simulink model "SvSDP_SimModel_FINAL_REV0"  (R2016b)
settings: Solver=ode3  StartTime=0  StopTime=15  FixedStep=T_sim  MaxStep=0.001  RelTol=1e-3  EnableMultiTasking=on
values from neighbouring files (symbols this model uses):
  A_A = pi/4*Dp^2    (= 0.00311724531052)    [par_SvSDP_SimModel_FINAL_REV0.m]
  A_B = pi/4*(Dp^2-Dr^2)    (= 0.00215513256036)    [par_SvSDP_SimModel_FINAL_REV0.m]
  beta_F = 7500e5    (= 750000000)    [par_SvSDP_SimModel_FINAL_REV0.m]
  Bs = 6480    [par_SvSDP_SimModel_FINAL_REV0.m]
  Drive_lim_max = 3000*pi/30    (= 314.159265359)    [par_SvSDP_SimModel_FINAL_REV0.m]
  Drive_lim_min = -3000*pi/30    (= -314.159265359)    [par_SvSDP_SimModel_FINAL_REV0.m]
  Drive_v_lim = 95e3*pi/30    (= 9948.37673637)    [par_SvSDP_SimModel_FINAL_REV0.m]
  dx_stribeck = 7e-3    (= 0.007)    [par_SvSDP_SimModel_FINAL_REV0.m]
  eta_air = 0.7e-2    (= 0.007)    [par_SvSDP_SimModel_FINAL_REV0.m]
  Fcs = 1740.8    [par_SvSDP_SimModel_FINAL_REV0.m]
  Fext = 20e3    (= 20000)    [par_SvSDP_SimModel_FINAL_REV0.m]
  Fss = Fcs+50    (= 1790.8)    [par_SvSDP_SimModel_FINAL_REV0.m]
  gammas = 1700    [par_SvSDP_SimModel_FINAL_REV0.m]
  I_nomK100 = 15.8    [par_SvSDP_SimModel_FINAL_REV0.m]
  Kad = H/(H+alpha)^2*abs(K_LpL)*10000    [par_SvSDP_SimModel_FINAL_REV0.m]
  kappa_air = 1.4    [par_SvSDP_SimModel_FINAL_REV0.m]
  kn_ad = A_A*(H+alpha)^2/(A_A^2*(H+alpha)^2+Bs*H*(K_LpL+Kad))    [par_SvSDP_SimModel_FINAL_REV0.m]
  Ms = 658    [par_SvSDP_SimModel_FINAL_REV0.m]
  pA_ini = Fext/A_A+alpha*pB_ini    (= 6485056.91477)    [par_SvSDP_SimModel_FINAL_REV0.m]
  pA_max = 500E5    (= 50000000)    [par_SvSDP_SimModel_FINAL_REV0.m]
  pA_min = 1E5    (= 100000)    [par_SvSDP_SimModel_FINAL_REV0.m]
  patm = 1.013e5    (= 101300)    [par_SvSDP_SimModel_FINAL_REV0.m]
  pB_ini = 1e5    (= 100000)    [par_SvSDP_SimModel_FINAL_REV0.m]
  pB_max = 500E5    (= 50000000)    [par_SvSDP_SimModel_FINAL_REV0.m]
  pB_min = 1E5    (= 100000)    [par_SvSDP_SimModel_FINAL_REV0.m]
  pset = 25e5    (= 2500000)    [par_SvSDP_SimModel_FINAL_REV0.m]
  pT = 1e5    (= 100000)    [par_SvSDP_SimModel_FINAL_REV0.m]
  Rs = 0.79    [par_SvSDP_SimModel_FINAL_REV0.m]
  tau_nomK100 = 28    [par_SvSDP_SimModel_FINAL_REV0.m]
  VAini = 0.36e-3    (= 0.00036)    [par_SvSDP_SimModel_FINAL_REV0.m]
  VBini = 0.54e-3    (= 0.00054)    [par_SvSDP_SimModel_FINAL_REV0.m]
  wn_m = 120*2*pi    (= 753.982236862)    [par_SvSDP_SimModel_FINAL_REV0.m]
  wn_V = 2*pi*21.22    (= 133.329192218)    [par_SvSDP_SimModel_FINAL_REV0.m]
  x_ini = 50e-3    (= 0.05)    [par_SvSDP_SimModel_FINAL_REV0.m]
  x_max = 700E-3    (= 0.7)    [par_SvSDP_SimModel_FINAL_REV0.m]
  x_min = 0E-3    (= 0)    [par_SvSDP_SimModel_FINAL_REV0.m]
  zeta_m = 0.50    (= 0.5)    [par_SvSDP_SimModel_FINAL_REV0.m]
  zeta_V = 1    [par_SvSDP_SimModel_FINAL_REV0.m]
undefined symbols (not defined in the file or in its folder): DAp_coeff, DBp_coeff, DCp_coeff, tauAp_coeff, tauBp_coeff, tauCp_coeff
libraries: cstblocks x2
settings Model: Creator=LS  LastModifiedBy=lsc
settings DataIOCC: LimitDataPoints=on  SaveFormat=Array  SignalLoggingSaveFormat=ModelDataLogs
settings OptimizationCC: BooleanDataType=off  ExpressionDepthLimit=2147483647  InitFltsAndDblsToZero=on  LifeSpan=inf
settings DebuggingCC: SaveWithParameterizedLinksMsg=none  UnderspecifiedInitializationDetection=Classic  MergeDetectMultiDrivingBlocksExec=none  SignalResolutionControl=TryResolveAllWithWarning  MultiTaskDSMMsg=warning  MultiTaskCondExecSysMsg=none  FcnCallInpInsideContextMsg=warning  StateNameClashWarn=warning  SFUnexpectedBacktrackingDiag=warning  SFNoUnconditionalDefaultTransitionDiag=warning  SFExecutionAtInitializationDiag=none
settings HardwareCC: ProdBitPerPointer=32  ProdBitPerSizeT=32  ProdBitPerPtrDiffT=32  ProdLargestAtomicFloat=None  ProdIntDivRoundTo=Undefined  ProdEndianess=Unspecified  ProdWordSize=32  ProdHWDeviceType=32-bit Generic  TargetBitPerPointer=64  TargetBitPerSizeT=64  TargetBitPerPtrDiffT=64  TargetLongLongMode=on  TargetIntDivRoundTo=Zero  TargetEndianess=LittleEndian  TargetWordSize=64  TargetHWDeviceType=MATLAB Host  ProdEqTarget=off
settings ModelReferenceCC: PropagateSignalLabelsOutOfModel=off
settings GRTTargetCC: TargetFcnLib=ansi_tfl_tmw.mat  TargetLangStandard=C89/C90 (ANSI)  GeneratePreprocessorConditionals=Disable all  CombineOutputUpdateFcns=off  GRTInterface=on
settings ConfigComp: CovMetricSettings=dw  CovHtmlReporting=on  CovSaveCumulativeToWorkspaceVar=on  CovSaveSingleToWorkspaceVar=on  CovExternalEMLEnable=off
settings ConfigurationSet: Description=SimMechanics 2G

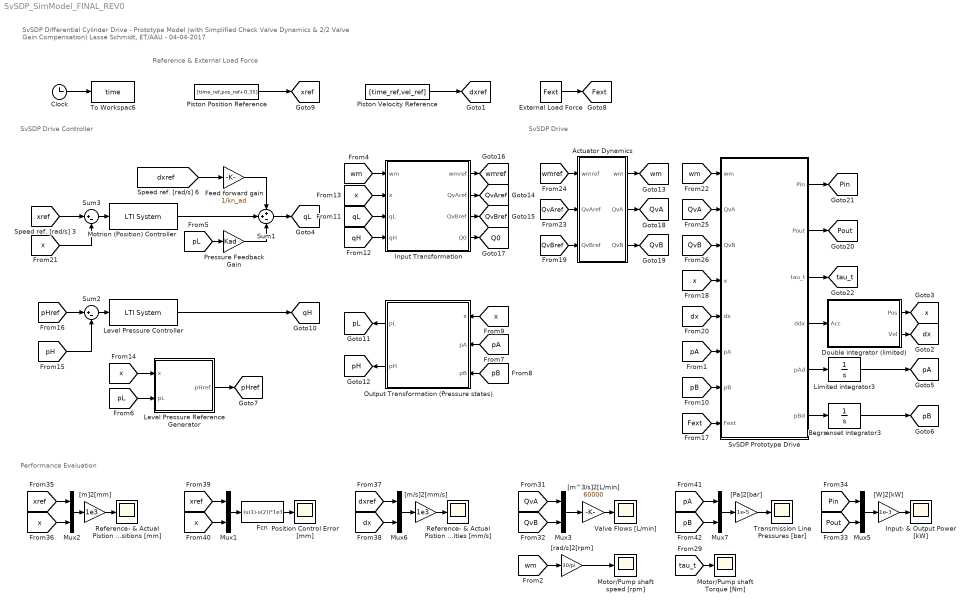
== system SvSDP_SimModel_FINAL_REV0 ==
  note: SvSDP Differential Cylinder Drive - Prototype Model (with Simplified Check Valve Dynamics & 2/2 Valve Gain Compensation) Lasse Schmidt, ET/AAU - 04-04-2017
  note: SvSDP Drive Controller
  note: SvSDP Drive
  note: Reference & External Load Force
  note: Performance Evaluation
  Actuator Dynamics : Subsystem
  Begrænset integrator3 : Integrator  InitialCondition=pB_ini  LimitOutput=on  UpperSaturationLimit=pB_max  LowerSaturationLimit=pB_min
  Clock : Clock
  Double integrator (limited) : Subsystem
  External Load Force : Constant  Value=Fext
  Fcn : Fcn  Expr=(u(1)-u(2))*1e3
  Feed forward gain : Gain  Gain=1/kn_ad
  Input Transformation : MATLAB Function  TreatAsAtomicUnit=on
  Input- & Output Power [kW] : Scope
  Level Pressure Controller : cstblocks/LTI System  sys=Gppi  IC=[]
  Level Pressure Reference Generator : MATLAB Function  TreatAsAtomicUnit=on
  Limited integrator3 : Integrator  InitialCondition=pA_ini  LimitOutput=on  UpperSaturationLimit=pA_max  LowerSaturationLimit=pA_min
  Motor/Pump shaft Torque [Nm] : Scope
  Motor/Pump shaft speed [rpm] : Scope
  Motrion (Position) Controller : cstblocks/LTI System  sys=Gmpi  IC=[]
  Mux{1..3,5..7} (6 alike) : Mux  Inputs=2
  Output Transformation (Pressure states) : MATLAB Function  TreatAsAtomicUnit=on
  Piston Position Reference : FromWorkspace  VariableName=[time_ref,pos_ref+0.35]  SampleTime=0
  Piston Velocity Reference : FromWorkspace  VariableName=[time_ref,vel_ref]  SampleTime=0
  Position Control Error [mm] : Scope
  Pressure Feedback Gain : Gain  Gain=Kad
  Reference- & Actual Pistion Positions [mm] : Scope
  Reference- & Actual Pistion Velocities [mm/s] : Scope
  Sum1 : Sum  Inputs=++-
  Sum2 : Sum  Inputs=|+-
  Sum3 : Sum  Inputs=|+-
  SvSDP Prototype Drive : MATLAB Function  TreatAsAtomicUnit=on
  To Workspac6 : ToWorkspace  VariableName=time  SampleTime=-1
  Transmission Line Pressures [bar] : Scope
  Valve Flows [L/min] : Scope
  "[Pa]2[bar]" : Gain  Gain=1e-5
  "[W]2[kW]" : Gain  Gain=1e-3
  "[m/s]2[mm/s]" : Gain  Gain=1e3
  "[m]2[mm]" : Gain  Gain=1e3
  "[m^3/s]2[L/min]" : Gain  Gain=60000
  "[rad/s]2[rpm]" : Gain  Gain=30/pi
  tag scope: Fext=global, Pin=global, Pout=global, Q0=global, QvA=global, QvAref=global, QvB=global, QvBref=global, dx=global, dxref=global, pA=global, pB=global, pH=global, pHref=global, pL=global, qH=global, qL=global, tau_t=global, wm=global, wmref=global, x=global, xref=global
  wires:
  Clock/1 -> To Workspac6/1
  Mux2/1 -> "[m]2[mm]"/1
  [xref] -> Mux2/1
  [x] -> Mux2/2
  SvSDP Prototype Drive/4(ddx) -> Double integrator (limited)/1(Acc)
  SvSDP Prototype Drive/6(pBd) -> Begrænset integrator3/1
  SvSDP Prototype Drive/5(pAd) -> Limited integrator3/1
  Limited integrator3/1 -> [pA]
  Begrænset integrator3/1 -> [pB]
  Double integrator (limited)/2(Vel) -> [dx]
  Double integrator (limited)/1(Pos) -> [x]
  [pB] -> SvSDP Prototype Drive/7(pB)
  [pA] -> SvSDP Prototype Drive/6(pA)
  [Fext] -> SvSDP Prototype Drive/8(Fext)
  [dx] -> SvSDP Prototype Drive/5(dx)
  [x] -> SvSDP Prototype Drive/4(x)
  Output Transformation (Pressure states)/1(pL) -> [pL]
  Output Transformation (Pressure states)/2(pH) -> [pH]
  [x] -> Output Transformation (Pressure states)/1(x)
  [pA] -> Output Transformation (Pressure states)/2(pA)
  [pB] -> Output Transformation (Pressure states)/3(pB)
  Input Transformation/2(QvAref) -> [QvAref]
  Input Transformation/3(QvBref) -> [QvBref]
  [x] -> Input Transformation/2(x)
  [qL] -> Input Transformation/3(qL)
  [qH] -> Input Transformation/4(qH)
  Input Transformation/1(wmref) -> [wmref]
  External Load Force/1 -> [Fext]
  [pL] -> Level Pressure Reference Generator/2(pL)
  [x] -> Level Pressure Reference Generator/1(x)
  Level Pressure Reference Generator/1(pHref) -> [pHref]
  [pHref] -> Sum2/1
  [pH] -> Sum2/2
  Sum2/1 -> Level Pressure Controller/1
  Sum1/1 -> [qL]
  [pL] -> Pressure Feedback Gain/1
  Sum3/1 -> Motrion (Position) Controller/1
  [x] -> Sum3/2
  Feed forward gain/1 -> Sum1/1
  Pressure Feedback Gain/1 -> Sum1/3
  [xref] -> Sum3/1
  [dxref] -> Feed forward gain/1
  Piston Velocity Reference/1 -> [dxref]
  Piston Position Reference/1 -> [xref]
  Mux3/1 -> "[m^3/s]2[L/min]"/1
  [QvB] -> Mux3/2
  [QvA] -> Mux3/1
  [wm] -> Input Transformation/1(wm)
  Input Transformation/4(Q0) -> [Q0]
  Motrion (Position) Controller/1 -> Sum1/2
  Level Pressure Controller/1 -> [qH]
  Actuator Dynamics/1(wm) -> [wm]
  [wmref] -> Actuator Dynamics/1(wmref)
  [QvAref] -> Actuator Dynamics/2(QvAref)
  [QvBref] -> Actuator Dynamics/3(QvBref)
  Actuator Dynamics/2(QvA) -> [QvA]
  Actuator Dynamics/3(QvB) -> [QvB]
  [wm] -> SvSDP Prototype Drive/1(wm)
  [QvA] -> SvSDP Prototype Drive/2(QvA)
  [QvB] -> SvSDP Prototype Drive/3(QvB)
  SvSDP Prototype Drive/3(tau_t) -> [tau_t]
  SvSDP Prototype Drive/2(Pout) -> [Pout]
  SvSDP Prototype Drive/1(Pin) -> [Pin]
  [tau_t] -> Motor/Pump shaft Torque [Nm]/1
  "[m^3/s]2[L/min]"/1 -> Valve Flows [L/min]/1
  Mux5/1 -> "[W]2[kW]"/1
  [Pin] -> Mux5/1
  [Pout] -> Mux5/2
  "[W]2[kW]"/1 -> Input- & Output Power [kW]/1
  "[m]2[mm]"/1 -> Reference- & Actual Pistion Positions [mm]/1
  Mux6/1 -> "[m/s]2[mm/s]"/1
  [dxref] -> Mux6/1
  [dx] -> Mux6/2
  "[m/s]2[mm/s]"/1 -> Reference- & Actual Pistion Velocities [mm/s]/1
  Mux1/1 -> Fcn/1
  [xref] -> Mux1/1
  [x] -> Mux1/2
  Fcn/1 -> Position Control Error [mm]/1
  Mux7/1 -> "[Pa]2[bar]"/1
  [pA] -> Mux7/1
  [pB] -> Mux7/2
  "[Pa]2[bar]"/1 -> Transmission Line Pressures [bar]/1
  [wm] -> "[rad/s]2[rpm]"/1
  "[rad/s]2[rpm]"/1 -> Motor/Pump shaft speed [rpm]/1

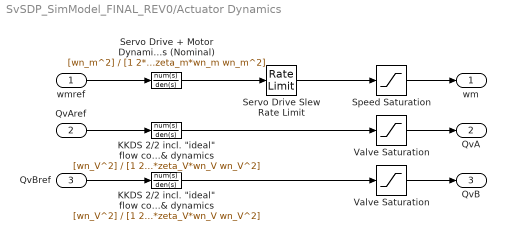
== system SvSDP_SimModel_FINAL_REV0/Actuator Dynamics ==
  wmref : Inport
  QvAref : Inport  Port=2
  QvBref : Inport  Port=3
  " KKDS 2/2 incl. \"ideal\" flow compensator & dynamics " : TransferFcn  Numerator=[wn_V^2]  Denominator=[1 2*zeta_V*wn_V wn_V^2]
  "KKDS 2/2 incl. \"ideal\" flow compensator & dynamics  " : TransferFcn  Numerator=[wn_V^2]  Denominator=[1 2*zeta_V*wn_V wn_V^2]
  Servo Drive + Motor Dynamics (Nominal) : TransferFcn  Numerator=[wn_m^2]  Denominator=[1 2*zeta_m*wn_m wn_m^2]
  Servo Drive Slew Rate Limit : RateLimiter  RisingSlewLimit=Drive_v_lim  FallingSlewLimit=-Drive_v_lim  SampleTimeMode=inherited
  Speed Saturation : Saturate  UpperLimit=Drive_lim_max  LowerLimit=Drive_lim_min
  Valve Saturation : Saturate  UpperLimit=inf  LowerLimit=0
  "Valve Saturation " : Saturate  UpperLimit=inf  LowerLimit=0
  wm : Outport
  QvA : Outport  Port=2
  QvB : Outport  Port=3
  wires:
  QvAref/1 -> "KKDS 2/2 incl. \"ideal\" flow compensator & dynamics  "/1
  QvBref/1 -> " KKDS 2/2 incl. \"ideal\" flow compensator & dynamics "/1
  wmref/1 -> Servo Drive + Motor Dynamics (Nominal)/1
  Servo Drive + Motor Dynamics (Nominal)/1 -> Servo Drive Slew Rate Limit/1
  "KKDS 2/2 incl. \"ideal\" flow compensator & dynamics  "/1 -> Valve Saturation/1
  " KKDS 2/2 incl. \"ideal\" flow compensator & dynamics "/1 -> "Valve Saturation "/1
  Valve Saturation/1 -> QvA/1
  Speed Saturation/1 -> wm/1
  "Valve Saturation "/1 -> QvB/1
  Servo Drive Slew Rate Limit/1 -> Speed Saturation/1

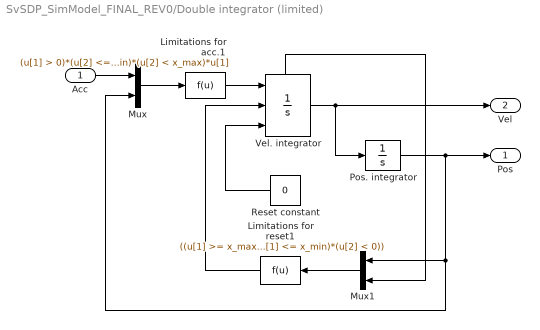
== system SvSDP_SimModel_FINAL_REV0/Double integrator (limited) ==
  Acc : Inport
  Limitations for acc.1 : Fcn  Expr=(u[1] > 0)*(u[2] <=x_min)*u[1]+(u[1] < 0)*(u[2] >=x_max)*u[1]+(u[2] > x_min)*(u[2] < x_max)*u[1]
  Limitations for reset1 : Fcn  Expr=((u[1] >= x_max)*(u[2] > 0)+(u[1] <= x_min)*(u[2] < 0))
  Mux : Mux  Inputs=2
  Mux1 : Mux  Inputs=2
  Pos. integrator : Integrator  InitialCondition=x_ini  LimitOutput=on  UpperSaturationLimit=x_max  LowerSaturationLimit=x_min
  Reset constant : Constant  Value=0
  Vel. integrator : Integrator  ExternalReset=level  InitialConditionSource=external  ShowStatePort=on
  Pos : Outport
  Vel : Outport  Port=2
  wires:
  Limitations for reset1/1 -> Vel. integrator/2
  Limitations for acc.1/1 -> Vel. integrator/1
  Pos. integrator/1 -> Mux1/1, Mux/2, Pos/1
  Vel. integrator/1 -> Pos. integrator/1, Vel/1
  Mux1/1 -> Limitations for reset1/1
  Reset constant/1 -> Vel. integrator/3
  Acc/1 -> Mux/1
  Mux/1 -> Limitations for acc.1/1
  Vel. integrator/State -> Mux1/2

== matlab function SvSDP_SimModel_FINAL_REV0/Output Transformation (Pressure states) ==
  data: x input; pL output; pH output; pA input; pB input; A_A parameter; A_B parameter; VAini parameter; VBini parameter; x_max parameter
function [pL,pH]  = fcn(x,pA,pB,A_A,A_B,VAini, VBini,x_max)

%% Output Transformation in SvSDP Drive Controller - Lasse Schmidt, ET/AAU - Date: 04-04-2017
%
% Area ratio
alpha = A_B/A_A;
% Instantaneous volumes
VA = VAini+A_A*x;
VB = VBini+(x_max-x)*A_B;
% Instantaneous volume ratio
rho = VB/VA;
% Instantaneous weighting factor H
H = rho/alpha;
% Virtual pressure states (from output transformation)
pL = pA-alpha*pB;
pH = pA+H*pB;
%% End

== matlab function SvSDP_SimModel_FINAL_REV0/SvSDP Prototype Drive ==
  data: Pin output; Pout output; tau_t output; ddx output; wm input; pAd output; QvA input; QvB input; x input; dx input; pA input; pB input; beta_F parameter; eta_air parameter; pBd output; patm parameter; kappa_air parameter; DAp_coeff parameter; DBp_coeff parameter; DCp_coeff parameter; Fcs parameter; Fss parameter; dx_stribeck parameter; gammas parameter; Bs parameter; A_A parameter; A_B parameter; Ms parameter; Fext input; VAini parameter; VBini parameter; x_max parameter; pT parameter; tauAp_coeff parameter; tauBp_coeff parameter; tauCp_coeff parameter; Rs parameter; I_nomK100 parameter; tau_nomK100 parameter
function [Pin,Pout,tau_t,ddx,pAd,pBd] = fcn(wm,QvA,QvB,x,dx,pA,pB,beta_F,eta_air,patm,kappa_air,DAp_coeff,DBp_coeff,DCp_coeff,Fcs,Fss,dx_stribeck,gammas,Bs,A_A,A_B,Ms,Fext,VAini, VBini,x_max,pT,tauAp_coeff, tauBp_coeff, tauCp_coeff,Rs, I_nomK100, tau_nomK100)

%% Speed-variable Switched Differential Pump (SvSDP) Cylinder Drive - Lasse Schmidt, ET/AAU - Date: 04-04-2017

%% Assumptions for SvSDP Drive Model
% - Flows from pressure compensated Bosch Rexroth KKDS 2/2 prop. valves are
%   assumed ideal, and furthermore ideally compensated such that QvA =
%   Gv(s)QvAref, QvB = Gv(s)QvBref is realized regardless of valve dynamics
% - Check valves are ideal such that flows through these are realized
%   instantaneously and without losses
% - As a result of the check valve assumption, the C-pump outlet pressure
%   is given by:
pC = (wm>=0)*pA+(wm<0)*pT;
%
%% Effective Bulk Modulii
% Effective bulkmodulus - A-line
beta_Ae = 1/(1/beta_F+1/(((1-eta_air)*(patm/(pA+patm))^(-1/kappa_air)/eta_air+1)*kappa_air*(pA+patm)));
% Effective bulkmodulus - B-line
beta_Be = 1/(1/beta_F+1/(((1-eta_air)*(patm/(pB+patm))^(-1/kappa_air)/eta_air+1)*kappa_air*(pB+patm)));
% Pump Flows - Bosch Rexroth AAAZPF-12-016/014/011
QpA = DAp_coeff(1)*wm + DAp_coeff(2)*(pA)+ DAp_coeff(3)*(pA)^2;
QpB = DBp_coeff(1)*wm + DBp_coeff(2)*(pB)+ DBp_coeff(3)*(pB)^2;
QpC = (wm>=0)*(DCp_coeff(1)*wm + DCp_coeff(2)*(pA)+ DCp_coeff(3)*(pA)^2)+(wm<0)*0;
% Friction Related to Cylinder & Load
Ff = (Fcs+(Fss-Fcs)*exp(-abs(dx)/dx_stribeck))*tanh(gammas*dx) + Bs*dx;
% Variable Volumes
VA = VAini+A_A*x;
VB = VBini+(x_max-x)*A_B;
%% Nonlinear State Equations
% A-line Pressure Dynamics
pAd = beta_Ae/VA*(QpA+QpC-A_A*dx-QvA);
% B-line Pressure Dynamics
pBd = beta_Be/VB*(A_B*dx-QpB-QvB);
% Motion Dynamics
ddx = 1/Ms*(pA*A_A-pB*A_B-Ff-Fext);
%% Auxiliary Properties
% Pump Torque - Bosch Rexroth AAAZPF-12-016/014/011
% Contribution from individual pumps
tau_Ap = tauAp_coeff(1)*sign(wm) + tauAp_coeff(2)*wm + tauAp_coeff(3)*sign(wm)*(pA-pT)+ tauAp_coeff(4)*(pA-pT);
tau_Bp = tauBp_coeff(1)*sign(wm) + tauBp_coeff(2)*wm + tauBp_coeff(3)*sign(wm)*(pB-pT)+ tauBp_coeff(4)*(pB-pT);
tau_Cp = tauCp_coeff(1)*sign(wm) + tauCp_coeff(2)*wm + tauCp_coeff(3)*sign(wm)*(pC-pT)+ tauCp_coeff(4)*(pC-pT);
% Total pump Torque
tau_t = tau_Ap + tau_Bp + tau_Cp;
% Input Power (Mechanical Including Ohmic Losses in PMSM Motor)
Pin = tau_t*wm+3*Rs*(tau_t*I_nomK100/tau_nomK100)^2;
% Output Power (Hydraulic via Cylinder Piston)
Pout = (A_A*pA-A_B*pB)*dx;
%% End

== matlab function SvSDP_SimModel_FINAL_REV0/Input Transformation ==
  data: wm input; wmref output; QvAref output; QvBref output; x input; qL input; qH input; VAini parameter; VBini parameter; x_max parameter; A_B parameter; A_A parameter; DAp_coeff parameter; DBp_coeff parameter; DCp_coeff parameter; Q0 output
function [wmref,QvAref,QvBref,Q0]  = fcn(wm,x,qL,qH,VAini, VBini,x_max,A_B, A_A,DAp_coeff, DBp_coeff, DCp_coeff)

%% Output Transformation in SvSDP Drive Controller - Lasse Schmidt, ET/AAU - Date: 04-04-2017
%
% Area ratio
alpha = A_B/A_A;
% Instantaneous volumes
VA = VAini+A_A*x;
VB = VBini+(x_max-x)*A_B;
% Instantaneous volume ratio
rho = VB/VA;
% Instantaneous vei9ghting factor H
H = rho/alpha;
% Directional dependent coefficient update
K_wA = (wm>=0)*(DAp_coeff(1) + DCp_coeff(1))+(wm<0)*DAp_coeff(1);
K_wB = DBp_coeff(1);
% Linearization coefficients 
Delta_Kw = K_wA - K_wB/alpha;
Lambda_Kw = K_wA + K_wB/H;
% References for actual (physical) inputs
wmref = (H+alpha)*qL/(Lambda_Kw*H);
QvAref = Delta_Kw*alpha*qL/(H*Lambda_Kw)-alpha*qH/(H+alpha)^2;
QvBref = Delta_Kw*alpha*qL/Lambda_Kw-H*alpha*qH/(H+alpha)^2;
% Virtual flow constraint (ideally Q0 = 0 should be satisfied)
Q0 = -QvAref+QvBref/H;
%% End

== matlab function SvSDP_SimModel_FINAL_REV0/Level Pressure Reference Generator ==
  data: pHref output; x input; pL input; VAini parameter; VBini parameter; x_max parameter; A_B parameter; A_A parameter; pset parameter
function pHref   = fcn(x,pL,VAini, VBini,x_max,A_B, A_A,pset)

%% Level Pressure Reference Generator in SvSDP Drive Controller - Lasse Schmidt, ET/AAU - Date: 04-04-2017
%
% Area ratio
alpha = A_B/A_A;
% Instantaneous volumes
VA = VAini+A_A*x;
VB = VBini+(x_max-x)*A_B;
% Instantaneous volume ratio
rho = VB/VA;
% Instantaneous vei9ghting factor H
H = rho/alpha;
% Load pressure switch condition
pLsw = pset*(1-alpha);
% Level pressure reference
pHref = (pL>=pLsw)*(pL+(H+alpha)*pset) + (pL<pLsw)*(-H/alpha*pL+(H+alpha)/alpha*pset);
%% End
